simulink model "DDMR_sim_pure_pursuit"  (R2022b)
settings: Solver=VariableStepAuto  StartTime=0.0  StopTime=10.0  RelTol=1e-3
undefined symbols (not defined in the file or in its folder): Cm, Jm, Kb, Kf, Kt, La, N, Ra
libraries: simulink x10
settings Model: Creator=CSPLAB  LastModifiedBy=CSPLAB

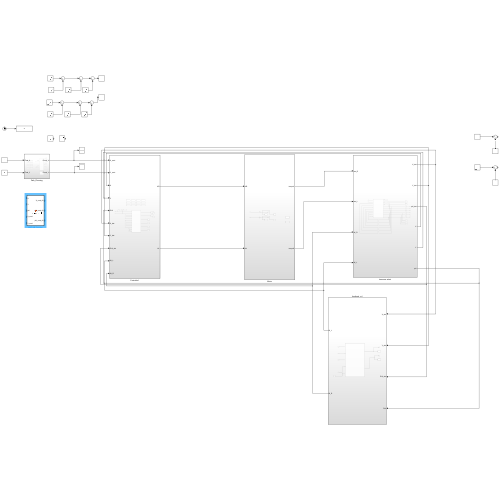
[thumbnail: Simulink's stored preview of the top-level diagram]
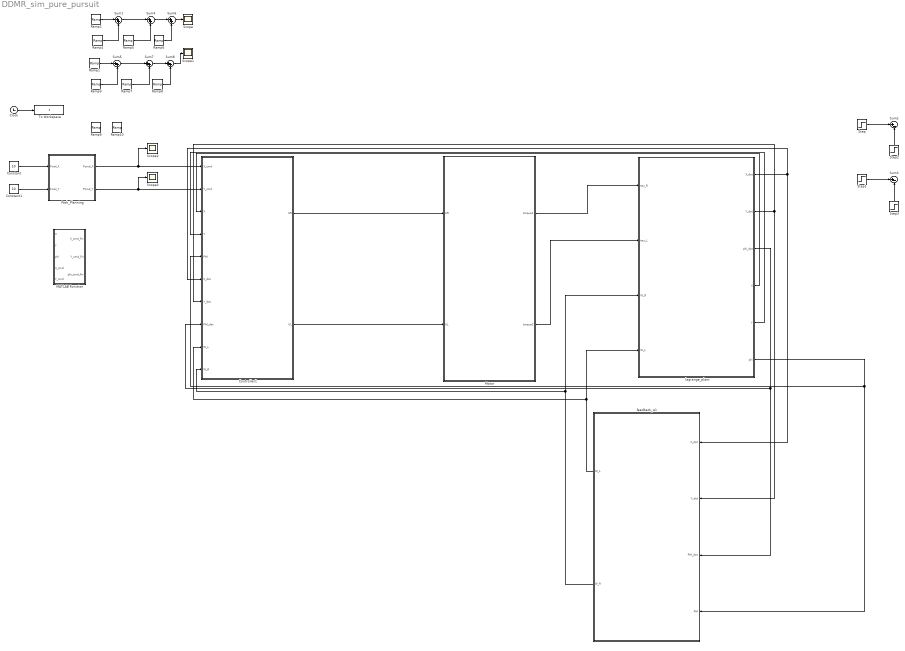
== system DDMR_sim_pure_pursuit ==
  Clock : Clock
  Constant : Constant  Value=10
  Constant1 : Constant  Value=10
  Controller1 : Subsystem
  MATLAB Function : MATLAB Function  TreatAsAtomicUnit=on
  Motor : Subsystem
  Path_Planning : Subsystem
  Ramp{1..2,9..10} (4 alike) : simulink/Sources/Ramp  slope=1  start=0  InitialOutput=0
  Ramp3 : simulink/Sources/Ramp  slope=-1  start=5  InitialOutput=0
  Ramp4 : simulink/Sources/Ramp  slope=-1  start=5  InitialOutput=0
  Ramp5 : simulink/Sources/Ramp  slope=-1  start=15  InitialOutput=0
  Ramp6 : simulink/Sources/Ramp  slope=1  start=20  InitialOutput=0
  Ramp7 : simulink/Sources/Ramp  slope=-1  start=15  InitialOutput=0
  Ramp8 : simulink/Sources/Ramp  slope=1  start=20  InitialOutput=0
  Scope{,1..3} (4 alike) : Scope
  Step : Step  Time=0  SampleTime=0
  Step1 : Step  Time=0  SampleTime=0
  Step2 : Step  Time=100  SampleTime=0
  Step3 : Step  Time=10  SampleTime=0
  Sum{1,4..8} (6 alike) : Sum  Inputs=|++
  Sum2 : Sum  Inputs=|+-
  Sum3 : Sum  Inputs=|+-
  To Workspace : ToWorkspace  VariableName=t  SampleTime=-1
  feedback_w1 : Subsystem
  lagrange_plant : Subsystem
  wires:
  Sum7/1 -> Sum8/1
  Motor/2(torque2) -> lagrange_plant/2(tau_L)
  Step/1 -> Sum2/1
  Constant1/1 -> Path_Planning/2(Final_Y)
  Ramp3/1 -> Sum5/2
  Ramp1/1 -> Sum5/1
  Constant/1 -> Path_Planning/1(Final_X)
  Ramp7/1 -> Sum7/2
  Sum8/1 -> Scope1/1
  Controller1/2(UL) -> Motor/2(UL)
  Sum1/1 -> Sum4/1
  Path_Planning/1(Pcmd_X) -> Scope2/1, Controller1/1(X_cmd)
  Step2/1 -> Sum2/2
  Motor/1(torque1) -> lagrange_plant/1(tau_R)
  Sum6/1 -> Scope/1
  lagrange_plant/3(phi_dot) -> Controller1/8(PHI_dot), feedback_w1/3(PHI_dot)
  Path_Planning/2(Pcmd_Y) -> Scope3/1, Controller1/2(Y_cmd)
  feedback_w1/1(W_L) -> Controller1/9(W_L), lagrange_plant/4(W_L)
  lagrange_plant/4(X) -> Controller1/3(X)
  Ramp5/1 -> Sum4/2
  lagrange_plant/5(Y) -> Controller1/4(Y)
  Controller1/1(UR) -> Motor/1(UR)
  lagrange_plant/6(phi) -> feedback_w1/4(PHI), Controller1/5(PHI)
  Sum5/1 -> Sum7/1
  Ramp8/1 -> Sum8/2
  Step3/1 -> Sum3/2
  Ramp4/1 -> Sum1/2
  feedback_w1/2(W_R) -> lagrange_plant/3(W_R), Controller1/10(W_R)
  Clock/1 -> To Workspace/1
  Ramp2/1 -> Sum1/1
  Sum4/1 -> Sum6/1
  Step1/1 -> Sum3/1
  Ramp6/1 -> Sum6/2
  lagrange_plant/2(Y_dot) -> Controller1/7(Y_dot), feedback_w1/2(Y_dot)
  lagrange_plant/1(X_dot) -> feedback_w1/1(X_dot), Controller1/6(X_dot)

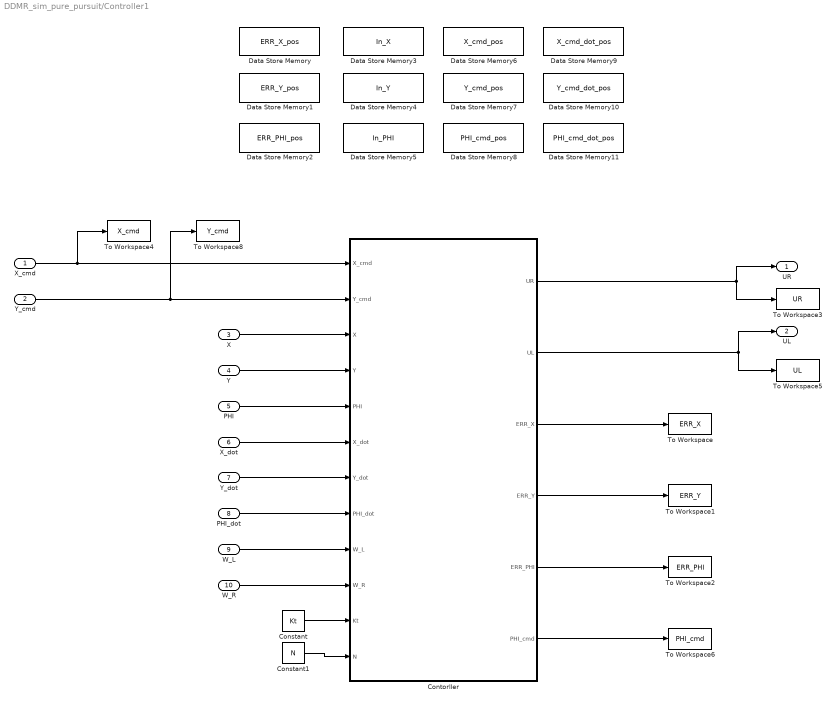
== system DDMR_sim_pure_pursuit/Controller1 ==
  X_cmd : Inport
  Y_cmd : Inport  Port=2
  X : Inport  Port=3
  Y : Inport  Port=4
  PHI : Inport  Port=5
  X_dot : Inport  Port=6
  Y_dot : Inport  Port=7
  PHI_dot : Inport  Port=8
  W_L : Inport  Port=9
  W_R : Inport  Port=10
  Constant : Constant  Value=Kt
  Constant1 : Constant  Value=N
  "Contorller " : MATLAB Function  TreatAsAtomicUnit=on
  Data Store Memory : DataStoreMemory  DataStoreName=ERR_X_pos  ReadBeforeWriteMsg=warning  WriteAfterWriteMsg=warning  WriteAfterReadMsg=warning  ShowAdditionalParam=off  OutDataTypeStr=double
  Data Store Memory1 : DataStoreMemory  DataStoreName=ERR_Y_pos  ReadBeforeWriteMsg=warning  WriteAfterWriteMsg=warning  WriteAfterReadMsg=warning  ShowAdditionalParam=off  OutDataTypeStr=double
  Data Store Memory10 : DataStoreMemory  DataStoreName=Y_cmd_dot_pos  ReadBeforeWriteMsg=warning  WriteAfterWriteMsg=warning  WriteAfterReadMsg=warning  ShowAdditionalParam=off  OutDataTypeStr=double
  Data Store Memory11 : DataStoreMemory  DataStoreName=PHI_cmd_dot_pos  ReadBeforeWriteMsg=warning  WriteAfterWriteMsg=warning  WriteAfterReadMsg=warning  ShowAdditionalParam=off  OutDataTypeStr=double
  Data Store Memory2 : DataStoreMemory  DataStoreName=ERR_PHI_pos  ReadBeforeWriteMsg=warning  WriteAfterWriteMsg=warning  WriteAfterReadMsg=warning  ShowAdditionalParam=off  OutDataTypeStr=double
  Data Store Memory3 : DataStoreMemory  DataStoreName=In_X  ReadBeforeWriteMsg=warning  WriteAfterWriteMsg=warning  WriteAfterReadMsg=warning  ShowAdditionalParam=off  OutDataTypeStr=double
  Data Store Memory4 : DataStoreMemory  DataStoreName=In_Y  ReadBeforeWriteMsg=warning  WriteAfterWriteMsg=warning  WriteAfterReadMsg=warning  ShowAdditionalParam=off  OutDataTypeStr=double
  Data Store Memory5 : DataStoreMemory  DataStoreName=In_PHI  ReadBeforeWriteMsg=warning  WriteAfterWriteMsg=warning  WriteAfterReadMsg=warning  ShowAdditionalParam=off  OutDataTypeStr=double
  Data Store Memory6 : DataStoreMemory  DataStoreName=X_cmd_pos  ReadBeforeWriteMsg=warning  WriteAfterWriteMsg=warning  WriteAfterReadMsg=warning  ShowAdditionalParam=off  OutDataTypeStr=double
  Data Store Memory7 : DataStoreMemory  DataStoreName=Y_cmd_pos  ReadBeforeWriteMsg=warning  WriteAfterWriteMsg=warning  WriteAfterReadMsg=warning  ShowAdditionalParam=off  OutDataTypeStr=double
  Data Store Memory8 : DataStoreMemory  DataStoreName=PHI_cmd_pos  ReadBeforeWriteMsg=warning  WriteAfterWriteMsg=warning  WriteAfterReadMsg=warning  ShowAdditionalParam=off  OutDataTypeStr=double
  Data Store Memory9 : DataStoreMemory  DataStoreName=X_cmd_dot_pos  ReadBeforeWriteMsg=warning  WriteAfterWriteMsg=warning  WriteAfterReadMsg=warning  ShowAdditionalParam=off  OutDataTypeStr=double
  To Workspace : ToWorkspace  VariableName=ERR_X  SampleTime=-1
  To Workspace1 : ToWorkspace  VariableName=ERR_Y  SampleTime=-1
  To Workspace2 : ToWorkspace  VariableName=ERR_PHI  SampleTime=-1
  To Workspace3 : ToWorkspace  VariableName=UR  SampleTime=-1
  To Workspace4 : ToWorkspace  VariableName=X_cmd  SampleTime=-1
  To Workspace5 : ToWorkspace  VariableName=UL  SampleTime=-1
  To Workspace6 : ToWorkspace  VariableName=PHI_cmd  SampleTime=-1
  To Workspace8 : ToWorkspace  VariableName=Y_cmd  SampleTime=-1
  UR : Outport  VectorParamsAs1DForOutWhenUnconnected=off
  UL : Outport  Port=2  VectorParamsAs1DForOutWhenUnconnected=off
  wires:
  "Contorller "/2(UL) -> To Workspace5/1, UL/1
  "Contorller "/1(UR) -> UR/1, To Workspace3/1
  W_R/1 -> "Contorller "/10(W_R)
  W_L/1 -> "Contorller "/9(W_L)
  PHI_dot/1 -> "Contorller "/8(PHI_dot)
  Y_dot/1 -> "Contorller "/7(Y_dot)
  X_dot/1 -> "Contorller "/6(X_dot)
  PHI/1 -> "Contorller "/5(PHI)
  Y/1 -> "Contorller "/4(Y)
  X/1 -> "Contorller "/3(X)
  Y_cmd/1 -> To Workspace8/1, "Contorller "/2(Y_cmd)
  X_cmd/1 -> To Workspace4/1, "Contorller "/1(X_cmd)
  Constant/1 -> "Contorller "/11(Kt)
  Constant1/1 -> "Contorller "/12(N)
  "Contorller "/5(ERR_PHI) -> To Workspace2/1
  "Contorller "/4(ERR_Y) -> To Workspace1/1
  "Contorller "/3(ERR_X) -> To Workspace/1
  "Contorller "/6(PHI_cmd) -> To Workspace6/1

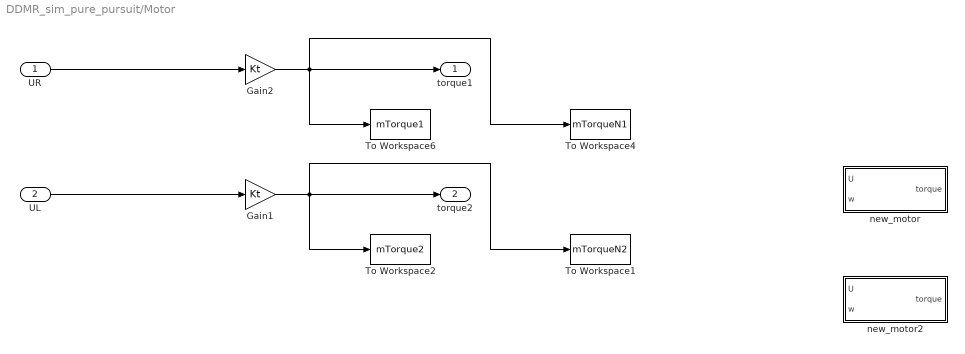
== system DDMR_sim_pure_pursuit/Motor ==
  UR : Inport
  UL : Inport  Port=2
  Gain1 : Gain  Gain=Kt
  Gain2 : Gain  Gain=Kt
  To Workspace1 : ToWorkspace  VariableName=mTorqueN2  SampleTime=-1
  To Workspace2 : ToWorkspace  VariableName=mTorque2  SampleTime=-1
  To Workspace4 : ToWorkspace  VariableName=mTorqueN1  SampleTime=-1
  To Workspace6 : ToWorkspace  VariableName=mTorque1  SampleTime=-1
  new_motor : Subsystem
  new_motor2 : Subsystem
  torque1 : Outport  VectorParamsAs1DForOutWhenUnconnected=off
  torque2 : Outport  Port=2  VectorParamsAs1DForOutWhenUnconnected=off
  wires:
  UR/1 -> Gain2/1
  Gain2/1 -> To Workspace6/1, To Workspace4/1, torque1/1
  Gain1/1 -> To Workspace2/1, To Workspace1/1, torque2/1
  UL/1 -> Gain1/1

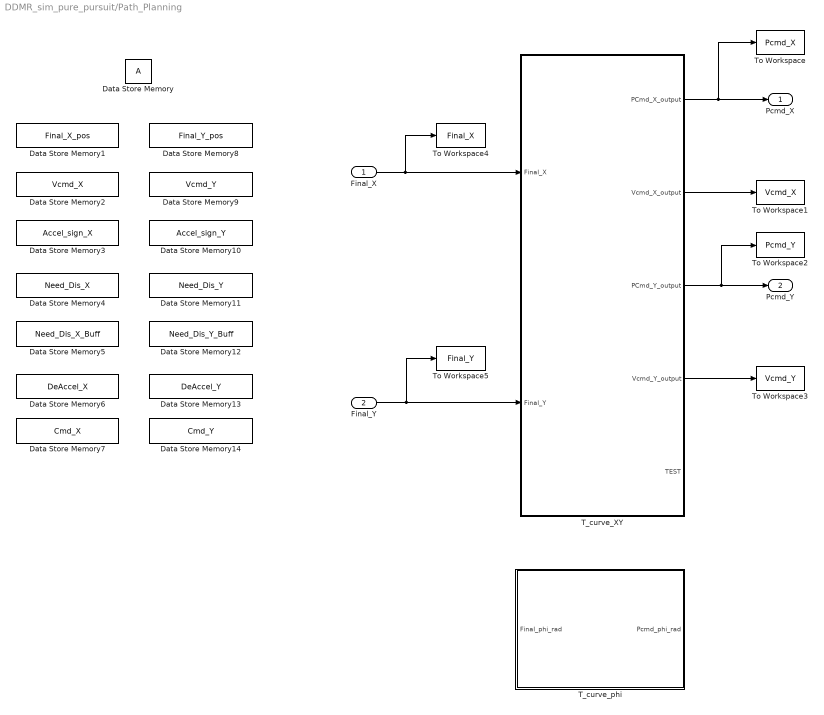
== system DDMR_sim_pure_pursuit/Path_Planning ==
  Final_X : Inport
  Final_Y : Inport  Port=2
  Data Store Memory : DataStoreMemory  ReadBeforeWriteMsg=warning  WriteAfterWriteMsg=warning  WriteAfterReadMsg=warning  ShowAdditionalParam=off  OutDataTypeStr=double
  Data Store Memory1 : DataStoreMemory  DataStoreName=Final_X_pos  ReadBeforeWriteMsg=warning  WriteAfterWriteMsg=warning  WriteAfterReadMsg=warning  ShowAdditionalParam=off  OutDataTypeStr=double
  Data Store Memory10 : DataStoreMemory  DataStoreName=Accel_sign_Y  ReadBeforeWriteMsg=warning  WriteAfterWriteMsg=warning  WriteAfterReadMsg=warning  ShowAdditionalParam=off  OutDataTypeStr=double
  Data Store Memory11 : DataStoreMemory  DataStoreName=Need_Dis_Y  ReadBeforeWriteMsg=warning  WriteAfterWriteMsg=warning  WriteAfterReadMsg=warning  ShowAdditionalParam=off  OutDataTypeStr=double
  Data Store Memory12 : DataStoreMemory  DataStoreName=Need_Dis_Y_Buff  ReadBeforeWriteMsg=warning  WriteAfterWriteMsg=warning  WriteAfterReadMsg=warning  ShowAdditionalParam=off  OutDataTypeStr=double
  Data Store Memory13 : DataStoreMemory  DataStoreName=DeAccel_Y  ReadBeforeWriteMsg=warning  WriteAfterWriteMsg=warning  WriteAfterReadMsg=warning  ShowAdditionalParam=off  OutDataTypeStr=double
  Data Store Memory14 : DataStoreMemory  DataStoreName=Cmd_Y  ReadBeforeWriteMsg=warning  WriteAfterWriteMsg=warning  WriteAfterReadMsg=warning  ShowAdditionalParam=off  OutDataTypeStr=double
  Data Store Memory2 : DataStoreMemory  DataStoreName=Vcmd_X  ReadBeforeWriteMsg=warning  WriteAfterWriteMsg=warning  WriteAfterReadMsg=warning  ShowAdditionalParam=off  OutDataTypeStr=double
  Data Store Memory3 : DataStoreMemory  DataStoreName=Accel_sign_X  ReadBeforeWriteMsg=warning  WriteAfterWriteMsg=warning  WriteAfterReadMsg=warning  ShowAdditionalParam=off  OutDataTypeStr=double
  Data Store Memory4 : DataStoreMemory  DataStoreName=Need_Dis_X  ReadBeforeWriteMsg=warning  WriteAfterWriteMsg=warning  WriteAfterReadMsg=warning  ShowAdditionalParam=off  OutDataTypeStr=double
  Data Store Memory5 : DataStoreMemory  DataStoreName=Need_Dis_X_Buff  ReadBeforeWriteMsg=warning  WriteAfterWriteMsg=warning  WriteAfterReadMsg=warning  ShowAdditionalParam=off  OutDataTypeStr=double
  Data Store Memory6 : DataStoreMemory  DataStoreName=DeAccel_X  ReadBeforeWriteMsg=warning  WriteAfterWriteMsg=warning  WriteAfterReadMsg=warning  ShowAdditionalParam=off  OutDataTypeStr=double
  Data Store Memory7 : DataStoreMemory  DataStoreName=Cmd_X  ReadBeforeWriteMsg=warning  WriteAfterWriteMsg=warning  WriteAfterReadMsg=warning  ShowAdditionalParam=off  OutDataTypeStr=double
  Data Store Memory8 : DataStoreMemory  DataStoreName=Final_Y_pos  ReadBeforeWriteMsg=warning  WriteAfterWriteMsg=warning  WriteAfterReadMsg=warning  ShowAdditionalParam=off  OutDataTypeStr=double
  Data Store Memory9 : DataStoreMemory  DataStoreName=Vcmd_Y  ReadBeforeWriteMsg=warning  WriteAfterWriteMsg=warning  WriteAfterReadMsg=warning  ShowAdditionalParam=off  OutDataTypeStr=double
  "T_curve_XY " : MATLAB Function  TreatAsAtomicUnit=on
  T_curve_phi : Subsystem
  To Workspace : ToWorkspace  VariableName=Pcmd_X  SampleTime=-1
  To Workspace1 : ToWorkspace  VariableName=Vcmd_X  SampleTime=-1
  To Workspace2 : ToWorkspace  VariableName=Pcmd_Y  SampleTime=-1
  To Workspace3 : ToWorkspace  VariableName=Vcmd_Y  SampleTime=-1
  To Workspace4 : ToWorkspace  VariableName=Final_X  SampleTime=-1
  To Workspace5 : ToWorkspace  VariableName=Final_Y  SampleTime=-1
  Pcmd_X : Outport  VectorParamsAs1DForOutWhenUnconnected=off
  Pcmd_Y : Outport  Port=2  VectorParamsAs1DForOutWhenUnconnected=off
  wires:
  Final_X/1 -> To Workspace4/1, "T_curve_XY "/1(Final_X)
  Final_Y/1 -> To Workspace5/1, "T_curve_XY "/2(Final_Y)
  "T_curve_XY "/1(PCmd_X_output) -> To Workspace/1, Pcmd_X/1
  "T_curve_XY "/3(PCmd_Y_output) -> To Workspace2/1, Pcmd_Y/1
  "T_curve_XY "/2(Vcmd_X_output) -> To Workspace1/1
  "T_curve_XY "/4(Vcmd_Y_output) -> To Workspace3/1

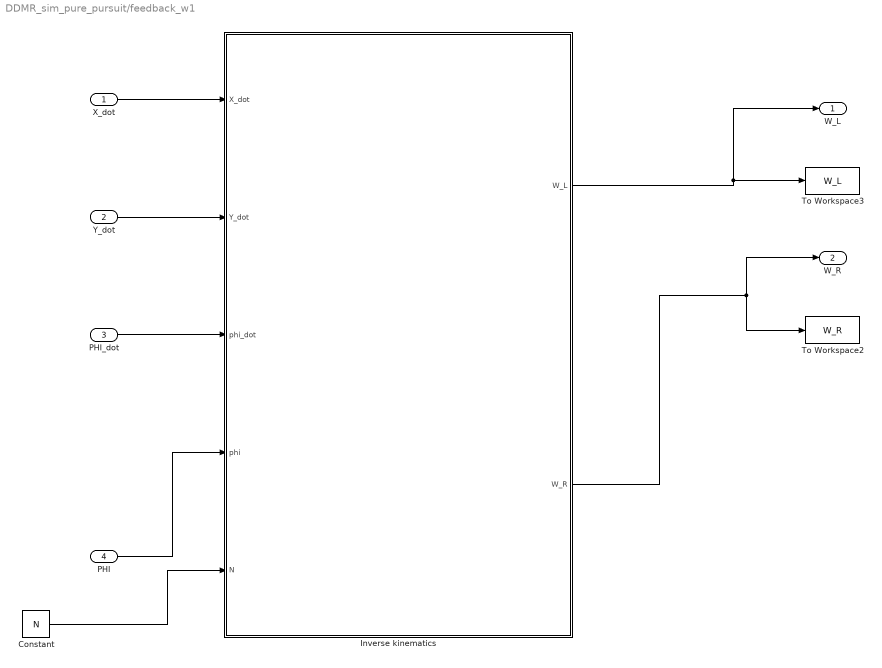
== system DDMR_sim_pure_pursuit/feedback_w1 ==
  X_dot : Inport
  Y_dot : Inport  Port=2
  PHI_dot : Inport  Port=3
  PHI : Inport  Port=4
  Constant : Constant  Value=N
  "Inverse kinematics " : MATLAB Function  TreatAsAtomicUnit=on
  To Workspace2 : ToWorkspace  VariableName=W_R  SampleTime=-1
  To Workspace3 : ToWorkspace  VariableName=W_L  SampleTime=-1
  W_L : Outport  VectorParamsAs1DForOutWhenUnconnected=off
  W_R : Outport  Port=2  VectorParamsAs1DForOutWhenUnconnected=off
  wires:
  PHI_dot/1 -> "Inverse kinematics "/3(phi_dot)
  PHI/1 -> "Inverse kinematics "/4(phi)
  Y_dot/1 -> "Inverse kinematics "/2(Y_dot)
  X_dot/1 -> "Inverse kinematics "/1(X_dot)
  "Inverse kinematics "/1(W_L) -> W_L/1, To Workspace3/1
  "Inverse kinematics "/2(W_R) -> W_R/1, To Workspace2/1
  Constant/1 -> "Inverse kinematics "/5(N)

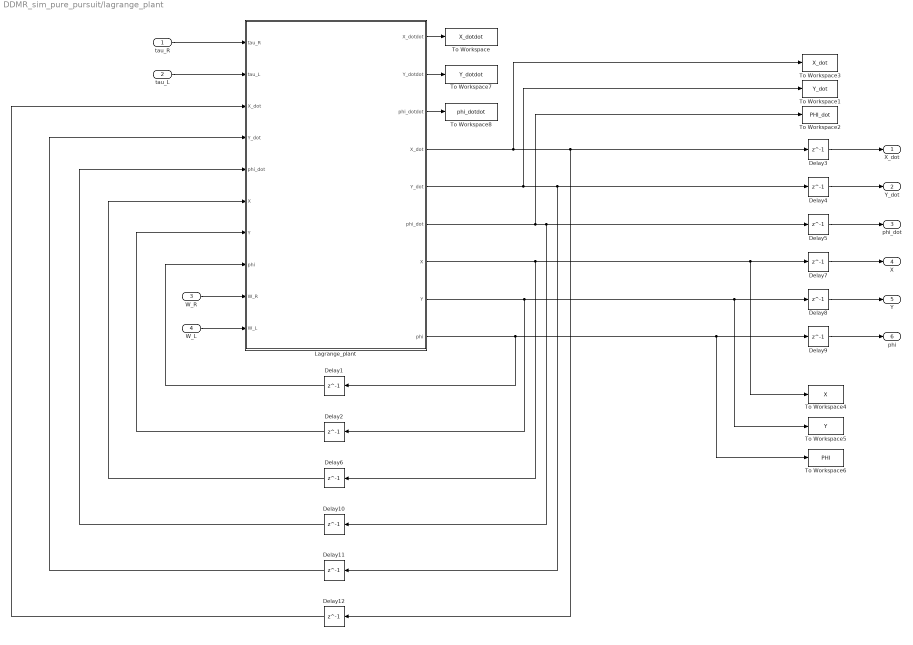
== system DDMR_sim_pure_pursuit/lagrange_plant ==
  tau_R : Inport
  tau_L : Inport  Port=2
  W_R : Inport  Port=3
  W_L : Inport  Port=4
  Delay{1..12} (12 alike) : Delay  DelayLength=1  InitialCondition=0
  Lagrange_plant : MATLAB Function  TreatAsAtomicUnit=on
  To Workspace : ToWorkspace  VariableName=X_dotdot  SampleTime=-1
  To Workspace1 : ToWorkspace  VariableName=Y_dot  SampleTime=-1
  To Workspace2 : ToWorkspace  VariableName=PHI_dot  SampleTime=-1
  To Workspace3 : ToWorkspace  VariableName=X_dot  SampleTime=-1
  To Workspace4 : ToWorkspace  VariableName=X  SampleTime=-1
  To Workspace5 : ToWorkspace  VariableName=Y  SampleTime=-1
  To Workspace6 : ToWorkspace  VariableName=PHI  SampleTime=-1
  To Workspace7 : ToWorkspace  VariableName=Y_dotdot  SampleTime=-1
  To Workspace8 : ToWorkspace  VariableName=phi_dotdot  SampleTime=-1
  X_dot : Outport
  Y_dot : Outport  Port=2
  phi_dot : Outport  Port=3
  X : Outport  Port=4
  Y : Outport  Port=5
  phi : Outport  Port=6
  wires:
  Delay3/1 -> X_dot/1
  W_L/1 -> Lagrange_plant/10(W_L)
  Lagrange_plant/8(Y) -> Delay2/1, To Workspace5/1, Delay8/1
  Lagrange_plant/4(X_dot) -> To Workspace3/1, Delay12/1, Delay3/1
  Delay10/1 -> Lagrange_plant/5("phi_dot ")
  Delay8/1 -> Y/1
  Delay12/1 -> Lagrange_plant/3("X_dot ")
  Delay9/1 -> phi/1
  Delay6/1 -> Lagrange_plant/6("X ")
  Lagrange_plant/9(phi) -> Delay1/1, To Workspace6/1, Delay9/1
  Lagrange_plant/5(Y_dot) -> To Workspace1/1, Delay11/1, Delay4/1
  Delay7/1 -> X/1
  Lagrange_plant/6(phi_dot) -> To Workspace2/1, Delay10/1, Delay5/1
  Delay1/1 -> Lagrange_plant/8("phi ")
  tau_R/1 -> Lagrange_plant/1(tau_R)
  W_R/1 -> Lagrange_plant/9(W_R)
  Lagrange_plant/7(X) -> Delay6/1, To Workspace4/1, Delay7/1
  Delay11/1 -> Lagrange_plant/4("Y_dot ")
  Delay4/1 -> Y_dot/1
  tau_L/1 -> Lagrange_plant/2(tau_L)
  Delay2/1 -> Lagrange_plant/7("Y ")
  Delay5/1 -> phi_dot/1
  Lagrange_plant/1(X_dotdot) -> To Workspace/1
  Lagrange_plant/2(Y_dotdot) -> To Workspace7/1
  Lagrange_plant/3(phi_dotdot) -> To Workspace8/1

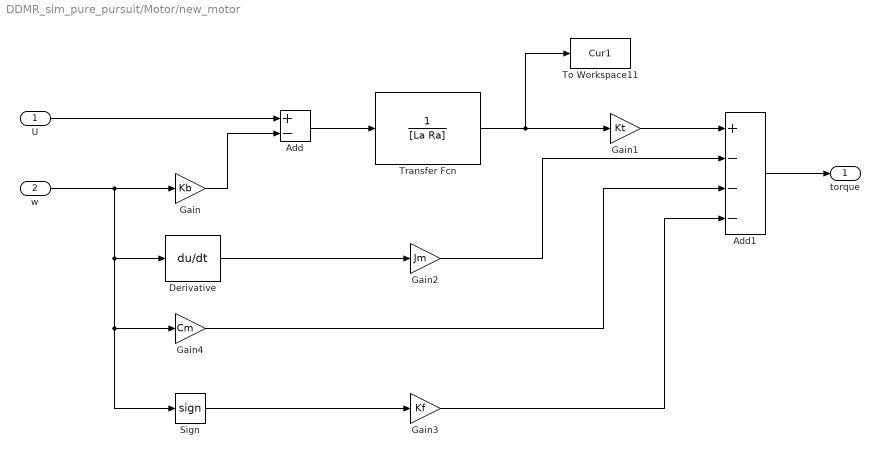
== system DDMR_sim_pure_pursuit/Motor/new_motor ==
  U : Inport
  w : Inport  Port=2
  Add : Sum  Inputs=+-
  Add1 : Sum  Inputs=+---
  Derivative : Derivative
  Gain : Gain  Gain=Kb
  Gain1 : Gain  Gain=Kt
  Gain2 : Gain  Gain=Jm
  Gain3 : Gain  Gain=Kf
  Gain4 : Gain  Gain=Cm
  Sign : Signum  ZeroCross=off
  To Workspace11 : ToWorkspace  VariableName=Cur1  SampleTime=-1
  Transfer Fcn : TransferFcn  Denominator=[La Ra]
  torque : Outport  VectorParamsAs1DForOutWhenUnconnected=off
  wires:
  Add1/1 -> torque/1
  Gain2/1 -> Add1/2
  Derivative/1 -> Gain2/1
  Gain1/1 -> Add1/1
  Gain4/1 -> Add1/3
  Gain/1 -> Add/2
  Transfer Fcn/1 -> To Workspace11/1, Gain1/1
  Sign/1 -> Gain3/1
  w/1 -> Sign/1, Gain4/1, Derivative/1, Gain/1
  U/1 -> Add/1
  Gain3/1 -> Add1/4
  Add/1 -> Transfer Fcn/1

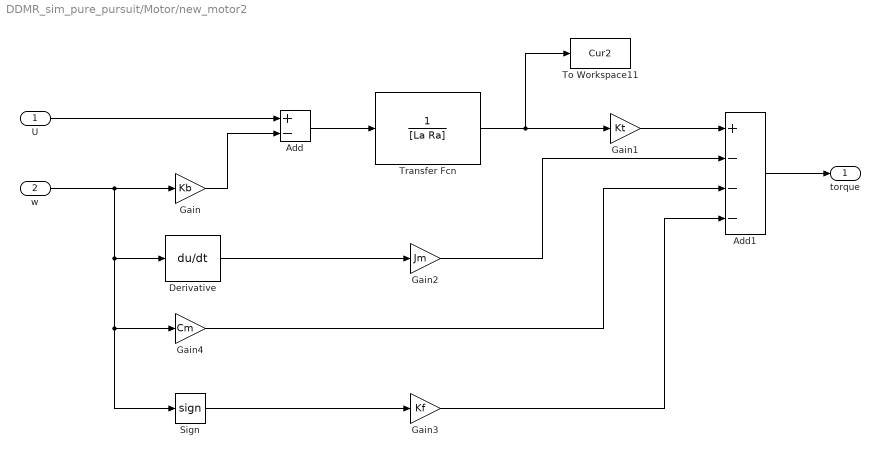
== system DDMR_sim_pure_pursuit/Motor/new_motor2 ==
  U : Inport
  w : Inport  Port=2
  Add : Sum  Inputs=+-
  Add1 : Sum  Inputs=+---
  Derivative : Derivative
  Gain : Gain  Gain=Kb
  Gain1 : Gain  Gain=Kt
  Gain2 : Gain  Gain=Jm
  Gain3 : Gain  Gain=Kf
  Gain4 : Gain  Gain=Cm
  Sign : Signum  ZeroCross=off
  To Workspace11 : ToWorkspace  VariableName=Cur2  SampleTime=-1
  Transfer Fcn : TransferFcn  Denominator=[La Ra]
  torque : Outport  VectorParamsAs1DForOutWhenUnconnected=off
  wires:
  Add1/1 -> torque/1
  Gain2/1 -> Add1/2
  Derivative/1 -> Gain2/1
  Gain1/1 -> Add1/1
  Gain4/1 -> Add1/3
  Add/1 -> Transfer Fcn/1
  Gain/1 -> Add/2
  Transfer Fcn/1 -> To Workspace11/1, Gain1/1
  Sign/1 -> Gain3/1
  w/1 -> Sign/1, Gain4/1, Derivative/1, Gain/1
  U/1 -> Add/1
  Gain3/1 -> Add1/4

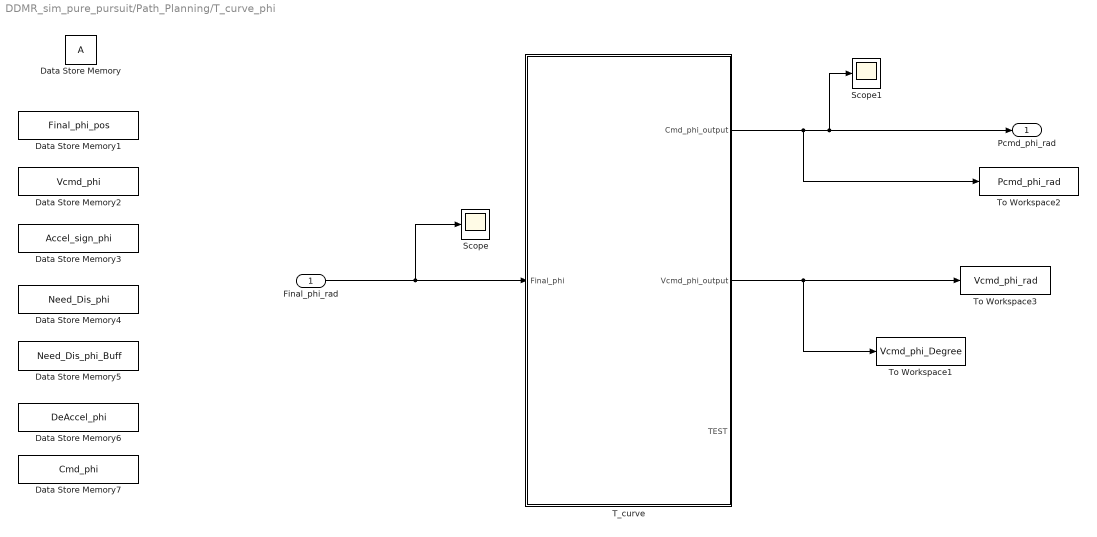
== system DDMR_sim_pure_pursuit/Path_Planning/T_curve_phi ==
  Final_phi_rad : Inport
  Data Store Memory : DataStoreMemory  ReadBeforeWriteMsg=warning  WriteAfterWriteMsg=warning  WriteAfterReadMsg=warning  ShowAdditionalParam=off  OutDataTypeStr=double
  Data Store Memory1 : DataStoreMemory  DataStoreName=Final_phi_pos  ReadBeforeWriteMsg=warning  WriteAfterWriteMsg=warning  WriteAfterReadMsg=warning  ShowAdditionalParam=off  OutDataTypeStr=double
  Data Store Memory2 : DataStoreMemory  DataStoreName=Vcmd_phi  ReadBeforeWriteMsg=warning  WriteAfterWriteMsg=warning  WriteAfterReadMsg=warning  ShowAdditionalParam=off  OutDataTypeStr=double
  Data Store Memory3 : DataStoreMemory  DataStoreName=Accel_sign_phi  ReadBeforeWriteMsg=warning  WriteAfterWriteMsg=warning  WriteAfterReadMsg=warning  ShowAdditionalParam=off  OutDataTypeStr=double
  Data Store Memory4 : DataStoreMemory  DataStoreName=Need_Dis_phi  ReadBeforeWriteMsg=warning  WriteAfterWriteMsg=warning  WriteAfterReadMsg=warning  ShowAdditionalParam=off  OutDataTypeStr=double
  Data Store Memory5 : DataStoreMemory  DataStoreName=Need_Dis_phi_Buff  ReadBeforeWriteMsg=warning  WriteAfterWriteMsg=warning  WriteAfterReadMsg=warning  ShowAdditionalParam=off  OutDataTypeStr=double
  Data Store Memory6 : DataStoreMemory  DataStoreName=DeAccel_phi  ReadBeforeWriteMsg=warning  WriteAfterWriteMsg=warning  WriteAfterReadMsg=warning  ShowAdditionalParam=off  OutDataTypeStr=double
  Data Store Memory7 : DataStoreMemory  DataStoreName=Cmd_phi  ReadBeforeWriteMsg=warning  WriteAfterWriteMsg=warning  WriteAfterReadMsg=warning  ShowAdditionalParam=off  OutDataTypeStr=double
  Scope : Scope
  Scope1 : Scope
  T_curve : MATLAB Function  TreatAsAtomicUnit=on
  To Workspace1 : ToWorkspace  VariableName=Vcmd_phi_Degree  SampleTime=-1
  To Workspace2 : ToWorkspace  VariableName=Pcmd_phi_rad  SampleTime=-1
  To Workspace3 : ToWorkspace  VariableName=Vcmd_phi_rad  SampleTime=-1
  Pcmd_phi_rad : Outport  VectorParamsAs1DForOutWhenUnconnected=off
  wires:
  Final_phi_rad/1 -> T_curve/1(Final_phi), Scope/1
  T_curve/2(Vcmd_phi_output) -> To Workspace3/1, To Workspace1/1
  T_curve/1(Cmd_phi_output) -> Scope1/1, Pcmd_phi_rad/1, To Workspace2/1

== matlab function DDMR_sim_pure_pursuit/Path_Planning/T_curve_XY  ==
  settings: updateMethod=DISCRETE  sampleTime=0.001
  data: A data_store_memory; PCmd_X_output output; Vcmd_X_output output; PCmd_Y_output output; Vcmd_Y_output output; Final_X input; TEST output; Final_X_pos data_store_memory; Vcmd_X data_store_memory; Accel_sign_X data_store_memory; Need_Dis_X data_store_memory; Need_Dis_X_Buff data_store_memory; DeAccel_X data_store_memory; Cmd_X data_store_memory; Final_Y input; Vcmd_Y data_store_memory; Final_Y_pos data_store_memory; Accel_sign_Y data_store_memory; Need_Dis_Y data_store_memory; Need_Dis_Y_Buff data_store_memory; DeAccel_Y data_store_memory; Cmd_Y data_store_memory
function [PCmd_X_output,Vcmd_X_output,PCmd_Y_output,Vcmd_Y_output,TEST]    = fcn(Final_X,Final_Y)

%==== Ver 2 =====
global A;
global Final_X_pos;
global Final_Y_pos;
global Vcmd_X;
global Vcmd_Y;
global Accel_sign_X;
global Accel_sign_Y;
global Need_Dis_X;
global Need_Dis_Y;
global Need_Dis_X_Buff;
global Need_Dis_Y_Buff;
global DeAccel_X;
global DeAccel_Y;
global Cmd_X;
global Cmd_Y;

%===== Parameter=====
Max_Accel = 1;
Max_Velocity = 1;
Pos_Standard = 0.1;
dt = 0.001;

%=== CHECK Final Change? ===
if(Final_X ~= Final_X_pos)
    Need_Dis_X = Final_X - Cmd_X;
    Need_Dis_X_Buff =0;
    DeAccel_X =0;
    
    %=== Direction Check ===
	if (Need_Dis_X >0)
        Accel_sign_X =  1;
	elseif (Need_Dis_X <0)
		Accel_sign_X = -1;
	else
		Accel_sign_X =  0;
	end
end

if(Final_Y ~= Final_Y_pos)
    Need_Dis_Y = Final_Y - Cmd_Y;
    Need_Dis_Y_Buff =0;
    DeAccel_Y =0;
    
    %=== Direction Check ===
	if (Need_Dis_Y >0)
        Accel_sign_Y =  1;
	elseif (Need_Dis_Y <0)
		Accel_sign_Y = -1;
	else
		Accel_sign_Y =  0;
	end
end

%===== Max Velocity Check =====
if( (abs(Need_Dis_X_Buff - Need_Dis_X ) > Pos_Standard) && (abs(Need_Dis_Y_Buff - Need_Dis_Y ) > Pos_Standard))
    Max_Velocity = 1.3;
else
    Max_Velocity = 2;
end



Detime_Y = abs(Vcmd_Y/Max_Accel);     
Detime_X = abs(Vcmd_X/Max_Accel);

%===== DeAccel Cehck =====
%===== X =====
     Buff = Need_Dis_X_Buff + Vcmd_X*Detime_X + 1/2*(-1*Accel_sign_X*Max_Accel)*Detime_X*Detime_X;
    
    if((Buff>Need_Dis_X) && (Accel_sign_X==1))
        DeAccel_X = 1;
    elseif ((Buff<Need_Dis_X) && (Accel_sign_X==-1))
        DeAccel_X = 1;
    else
        DeAccel_X = 0;
    end
%===== Y =====    
         Buff = Need_Dis_Y_Buff + Vcmd_Y*Detime_Y + 1/2*(-1*Accel_sign_Y*Max_Accel)*Detime_Y*Detime_Y;
    
    if((Buff>Need_Dis_Y) && (Accel_sign_Y==1))
        DeAccel_Y = 1;
    elseif ((Buff<Need_Dis_Y) && (Accel_sign_Y==-1))
        DeAccel_Y = 1;
    else
        DeAccel_Y = 0;
    end
    
%===== Vel Cal =====
%===== X =====
if(DeAccel_X ==0)
    Vcmd_X = Vcmd_X + Accel_sign_X * Max_Accel*dt;
elseif(DeAccel_X ==1) 
    Vcmd_X = Vcmd_X - Accel_sign_X * Max_Accel*dt;
    Buff = Vcmd_X *Accel_sign_X;
    if(Buff<0)
    Vcmd_X = 0;
    end
end
%===== Y =====
if(DeAccel_Y ==0)
    Vcmd_Y = Vcmd_Y + Accel_sign_Y * Max_Accel*dt;
elseif(DeAccel_Y ==1) 
    Vcmd_Y = Vcmd_Y - Accel_sign_Y * Max_Accel*dt;
    Buff = Vcmd_Y *Accel_sign_Y;
    if(Buff<0)
    Vcmd_Y = 0;
    end
end

%===== Max Vel Check =====
%=== X ===
if(Vcmd_X > Max_Velocity)
    Vcmd_X = Max_Velocity;
elseif (Vcmd_X < -Max_Velocity)
    Vcmd_X = -Max_Velocity;
end
%=== Y ===
if(Vcmd_Y > Max_Velocity)
    Vcmd_Y = Max_Velocity;
elseif (Vcmd_Y < -Max_Velocity)
    Vcmd_Y = -Max_Velocity;
end


Cmd_X = Cmd_X + Vcmd_X * dt;
Cmd_Y = Cmd_Y + Vcmd_Y * dt;

Need_Dis_X_Buff = Need_Dis_X_Buff + Vcmd_X*dt;
Need_Dis_Y_Buff = Need_Dis_Y_Buff + Vcmd_Y*dt;

Final_X_pos = Final_X;
Final_Y_pos = Final_Y;

%===== Output =====
PCmd_X_output  = Cmd_X;
PCmd_Y_output  = Cmd_Y;

Vcmd_X_output = Vcmd_X;
Vcmd_Y_output = Vcmd_Y;

A = A+1;
TEST =A;

== matlab function DDMR_sim_pure_pursuit/lagrange_plant/Lagrange_plant ==
  data: tau_R input; X_dotdot output; tau_L input; X_dot input; Y_dot input; phi_dot input; X input; Y input; phi input; W_R input; W_L input; Y_dotdot output; phi_dotdot output; X_dot output; Y_dot output; phi_dot output; X output; Y output; phi output
function [X_dotdot,Y_dotdot,phi_dotdot,X_dot,Y_dot,phi_dot,X,Y,phi] = fcn(tau_R,tau_L,X_dot,Y_dot,phi_dot,X,Y,phi,W_R,W_L)
%#codegen

%%
%parameter
dt = 0.001;

%car parameter
%重量單位:kg 
%長度單位:m

%body
m_b = 1200; 
d_b = 0.81;
L_b = 1.069; 
I_zb = 1/12*m_b*(d_b^2+L_b^2);
%wheel
m_w = 10; 
R = 0.09;
L = 0.4;
I_yw = m_w*R^2/2;
d = 0;
I_zw = m_w*(L^2 + d^2);


%dynamic model
BUFF_POSI = 2*I_yw*+R^2*m_b+2*R^2*m_w;
BUFF_ANGLE = -I_yw*L^2+2*I_zb*R^2+4*I_zw*R^2+L^2*R^2*m_w;

X_dotdot = R*cos(phi)*(tau_L+tau_R)/BUFF_POSI;
Y_dotdot = R*sin(phi)*(tau_L+tau_R)/BUFF_POSI;
phi_dotdot = R*L*(tau_L-tau_R)/BUFF_ANGLE;

X_dot = X_dot + X_dotdot*dt;
Y_dot = Y_dot + Y_dotdot*dt;
phi_dot = phi_dot + phi_dotdot*dt;

X = X + X_dot*dt;
Y = Y + Y_dot*dt;
phi = phi + phi_dot*dt;

== matlab function DDMR_sim_pure_pursuit/feedback_w1/Inverse kinematics  ==
  settings: updateMethod=DISCRETE  sampleTime=0.001
  data: X_dot input; Y_dot input; phi_dot input; W_L output; W_R output; phi input; N input
function [W_L,W_R]  = fcn(X_dot,Y_dot,phi_dot,phi,N)
%#codegen




% ===== Parameter =====
L = 0.4;
R = 0.09;

W_R = (cos(phi)/R*X_dot + sin(phi)/R*Y_dot + L/(2*R)*phi_dot)/N;
W_L = (cos(phi)/R*X_dot + sin(phi)/R*Y_dot - L/(2*R)*phi_dot)/N;

== matlab function DDMR_sim_pure_pursuit/Controller1/Contorller  ==
  settings: updateMethod=DISCRETE  sampleTime=0.001
  data: X_cmd input; UR output; UL output; Y_cmd input; X input; Y input; PHI input; X_dot input; Y_dot input; PHI_dot input; W_L input; W_R input; ERR_X_pos data_store_memory; ERR_Y_pos data_store_memory; ERR_PHI_pos data_store_memory; In_X data_store_memory; In_Y data_store_memory; In_PHI data_store_memory; X_cmd_pos data_store_memory; Y_cmd_pos data_store_memory; PHI_cmd_pos data_store_memory; X_cmd_dot_pos data_store_memory; Y_cmd_dot_pos data_store_memory; PHI_cmd_dot_pos data_store_memory; ERR_X output; ERR_Y output; ERR_PHI output; Kt input; N input; PHI_cmd output
function [UR,UL,ERR_X,ERR_Y,ERR_PHI,PHI_cmd]  = fcn(X_cmd,Y_cmd,X,Y,PHI,X_dot,Y_dot,PHI_dot,W_L,W_R,Kt,N)
%#codegen

global In_X
global In_Y
global In_PHI
global ERR_X_pos
global ERR_Y_pos
global ERR_PHI_pos
global X_cmd_pos
global Y_cmd_pos
global PHI_cmd_pos
global X_cmd_dot_pos
global Y_cmd_dot_pos
global PHI_cmd_dot_pos


%parameter
dt = 0.001;
PHI_cmd = 0;
%car parameter
%重量單位:kg 
%長度單位:m

%body
m_b = 1200; 
d_b = 0.81;
L_b = 1.069; 
I_zb = 1/12*m_b*(d_b^2+L_b^2);
%wheel
m_w = 10; 
R = 0.09;
L = 0.4;
I_yw = m_w*R^2/2;
d = 0;
I_zw = m_w*(L^2 + d^2);
X_dir = 0;
% %=== Motor ===
% Ra = 0.38;
% Kt = 28.6*10^-3;
% Kb = Kt;
% 
% %=== Gear ===
% N = 14;

%=== Sat ===
MaxU = 24;

dt = 0.001;
%===== Command =====%

%===== Controller =====
Kp = 9550;
Ki = 65;
Kd = 45;

Kp_phi = 120;
kd_phi = 0;
ki_phi = 20;

ERR_X   = X_cmd   - X;
ERR_Y   = Y_cmd   - Y;


PHI_cmd = abs(atan2d(ERR_Y,ERR_X));
if(PHI_cmd == 180)
    PHI_cmd = 0
end

% if(ERR_X == 0)
%     if(ERR_Y > 0)
%         PHI_cmd = 90;%degree
%     else if(ERR_Y < 0)
%         PHI_cmd = 270;
%     end
%     end
% end
% 
% if(ERR_Y == 0)
%     if(ERR_X > 0)
%         PHI_cmd = 0;%degree
%     else if(ERR_Y < 0)
%         PHI_cmd = 180;
%     end
%     end
% end
% if(ERR_X > 0 && ERR_Y > 0)
%     PHI_cmd = atan(ERR_Y/ERR_X);%degree
% else if(ERR_X < 0 && ERR_Y < 0)
%     PHI_cmd = atan(ERR_Y/ERR_X) + 180;%degree
% else if(ERR_X < 0 && ERR_Y > 0)
%     PHI_cmd = atan(ERR_Y/ERR_X);
% else if(ERR_X > 0 && ERR_Y < 0)
%     PHI_cmd = atan(ERR_Y/ERR_X) + 180;
% end        
% end
% end
% end  
ERR_PHI = PHI_cmd - PHI;
% ===== X =====
X_cmd_dot = (X_cmd - X_cmd_pos)/dt ;
X_cmd_dotdot = (X_cmd_dot - X_cmd_dot_pos)/dt;

Pr_X = Kp*ERR_X;
In_X = In_X + Ki*ERR_X*dt;
Di_X = Kd*(ERR_X-ERR_X_pos)/dt;

X_all =  X_cmd_dotdot + Pr_X + In_X + Di_X ;

% ===== Y =====
Y_cmd_dot = (Y_cmd - Y_cmd_pos)*dt ;
Y_cmd_dotdot = (Y_cmd_dot - Y_cmd_dot_pos)/dt;

Pr_Y = Kp*ERR_Y;
In_Y = In_Y + Ki*ERR_Y*dt;
Di_Y = Kd*(ERR_Y-ERR_Y_pos)/dt;

Y_all = Y_cmd_dotdot + Pr_Y + In_Y + Di_Y ;

% % ===== PHI =====
PHI_cmd_dot = (PHI_cmd - PHI_cmd_pos)/dt ;
PHI_cmd_dotdot = (PHI_cmd_dot - PHI_cmd_dot_pos)/dt;

Pr_PHI = Kp_phi*ERR_PHI;
In_PHI = In_PHI + ki_phi*ERR_PHI*dt;
Di_PHI = kd_phi*(ERR_PHI-ERR_PHI_pos)/dt;

PHI_all = PHI_cmd_dotdot + Pr_PHI + In_PHI + Di_PHI;


% ===== TQC =====
BUFF_POSI = 2*I_yw*+R^2*m_b+2*R^2*m_w;
BUFF_ANGLE = -I_yw*L^2+2*I_zb*R^2+4*I_zw*R^2+L^2*R^2*m_w;

% === MR ====
Buff_X   =  cos(PHI)/(2*R)*BUFF_POSI;
Buff_Y   =  sin(PHI)/(2*R)*BUFF_POSI;
Buff_PHI =  -BUFF_ANGLE/(2*L*R);

TQC1 = (Buff_X*X_all + Buff_Y*Y_all + Buff_PHI*PHI_all)/N;

% === ML ====
Buff_X   =  cos(PHI)/(2*R)*BUFF_POSI;
Buff_Y   =  sin(PHI)/(2*R)*BUFF_POSI;
Buff_PHI =  BUFF_ANGLE/(2*L*R);

TQC2 = (Buff_X*X_all + Buff_Y*Y_all + Buff_PHI*PHI_all)/N;





% TQC_to_Uc

UR = TQC1/(Kt*N);
UL = TQC2/(Kt*N);

% 
% if ( abs(UR)>MaxU )
%     UR =sign(UR)*MaxU;
% end
% 
% if ( abs(UL)>MaxU )
%     UL =sign(UL)*MaxU;
% end
% 




%===== Recorder =====
X_cmd_pos = X_cmd;
Y_cmd_pos = Y_cmd;
PHI_cmd_pos = PHI_cmd;

X_cmd_dot_pos = X_cmd_dot;
Y_cmd_dot_pos = Y_cmd_dot;
PHI_cmd_dot_pos = PHI_cmd_dot;

ERR_X_pos   = ERR_X;
ERR_Y_pos   = ERR_Y;
ERR_PHI_pos = ERR_PHI;

== matlab function DDMR_sim_pure_pursuit/Path_Planning/T_curve_phi/T_curve ==
  settings: updateMethod=DISCRETE  sampleTime=0.001
  data: A data_store_memory; Cmd_phi_output output; Vcmd_phi_output output; Final_phi input; TEST output; Final_phi_pos data_store_memory; Vcmd_phi data_store_memory; Accel_sign_phi data_store_memory; Need_Dis_phi data_store_memory; Need_Dis_phi_Buff data_store_memory; DeAccel_phi data_store_memory; Cmd_phi data_store_memory
function [Cmd_phi_output,Vcmd_phi_output,TEST]    = fcn(Final_phi)

%==== Ver 2 =====

global A;
global Final_phi_pos;
global Vcmd_phi;
global Accel_sign_phi;
global Need_Dis_phi;
global Need_Dis_phi_Buff;
global DeAccel_phi;
global Cmd_phi;

%===== Parameter=====
Max_Accel = pi/4;
Max_Velocity = pi/4;
Pos_Standard = 0.1;
dt = 0.001;

%=== CHECK Final Change? ===
if(Final_phi ~= Final_phi_pos)
    Need_Dis_phi = Final_phi - Cmd_phi;
    Need_Dis_phi_Buff =0;
    DeAccel_phi =0;
    
    %=== Direction Check ===
	if (Need_Dis_phi >0)
        Accel_sign_phi =  1;
	elseif (Need_Dis_phi <0)
		Accel_sign_phi = -1;
	else
		Accel_sign_phi =  0;
	end
end
    
Detime_phi = abs(Vcmd_phi/Max_Accel);

%===== DeAccel Cehck =====
     Buff = Need_Dis_phi_Buff + Vcmd_phi*Detime_phi + 1/2*(-1*Accel_sign_phi*Max_Accel)*Detime_phi*Detime_phi;
    
    if((Buff>Need_Dis_phi) && (Accel_sign_phi==1))
        DeAccel_phi = 1;
    elseif ((Buff<Need_Dis_phi) && (Accel_sign_phi==-1))
        DeAccel_phi = 1;
    else
        DeAccel_phi = 0;
    end
    
%===== Vel Cal =====
if(DeAccel_phi ==0)
    Vcmd_phi = Vcmd_phi + Accel_sign_phi * Max_Accel*dt;
elseif(DeAccel_phi ==1) 
    Vcmd_phi = Vcmd_phi - Accel_sign_phi * Max_Accel*dt;
    Buff = Vcmd_phi *Accel_sign_phi;
    if(Buff<0)
    Vcmd_phi = 0;
    end
end

%===== Max Vel Check =====

if(Vcmd_phi > Max_Velocity)
    Vcmd_phi = Max_Velocity;
elseif (Vcmd_phi < -Max_Velocity)
    Vcmd_phi = -Max_Velocity;
end


Cmd_phi = Cmd_phi + Vcmd_phi * dt;
Need_Dis_phi_Buff = Need_Dis_phi_Buff + Vcmd_phi*dt;
Final_phi_pos = Final_phi;

%===== Output =====
Cmd_phi_output  = Cmd_phi ;
Vcmd_phi_output = Vcmd_phi;

A = A+1;
TEST =A;

== matlab function DDMR_sim_pure_pursuit/MATLAB Function ==
  data: X input; X_cmd_fin output; Y_cmd_fin output; Y input; phi input; X_cmd input; Y_cmd input; phi_cmd_fin output
function [X_cmd_fin,Y_cmd_fin,phi_cmd_fin] = pure_purpursuit(X,Y,phi,X_cmd,Y_cmd)

    ERR_X = X_cmd - X;
    ERR_Y = Y_cmd - Y;
    ERR_phi = phi_cmd - phi;
